simulink model "obs_servo_reduced"  (R2022a)
settings: Solver=VariableStepAuto  StartTime=0.0  StopTime=20  RelTol=1e-3
values from neighbouring files (symbols this model uses):
  A = [0 0 0 1 0 0 ... (first row only)    [main.m]
  Aroi = inv(Aro)    [main.m]
  B = [0 0 ... (first row only)    [main.m]
  C = [1 0 0 0 0 0 ... (first row only)    [main.m]
  D1 = [-3.6,0,0 ... (first row only)    [main.m]
  Eo = Tr*B    [main.m]
  Go = eye(3)    [main.m]
  ka5 = real(inv(R)*Ba5'*P2)    [main.m]
  ysp = -0.1*C*inv(A)*B*[-0.5+(a-b)/20;0.1+(b-c/(a+d+10))]    [main.m]
settings Model: Creator=wyton  LastModifiedBy=dzsgy
settings SolverCC: AlgebraicLoopSolver=TrustRegion
settings DebuggingCC: UnconnectedInputMsg=warning  UnconnectedOutputMsg=warning  UnconnectedLineMsg=warning  SFMachineParentedDataDiag=warning

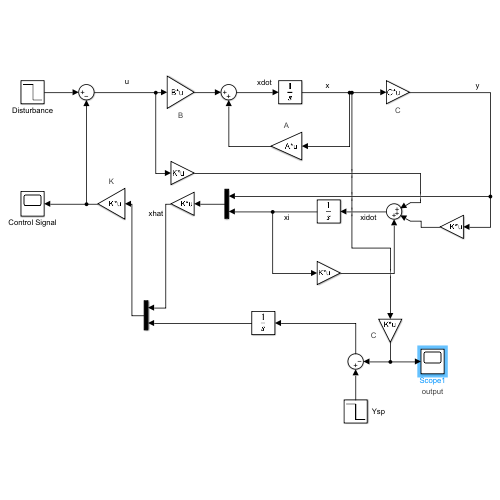
[thumbnail: Simulink's stored preview of the top-level diagram]
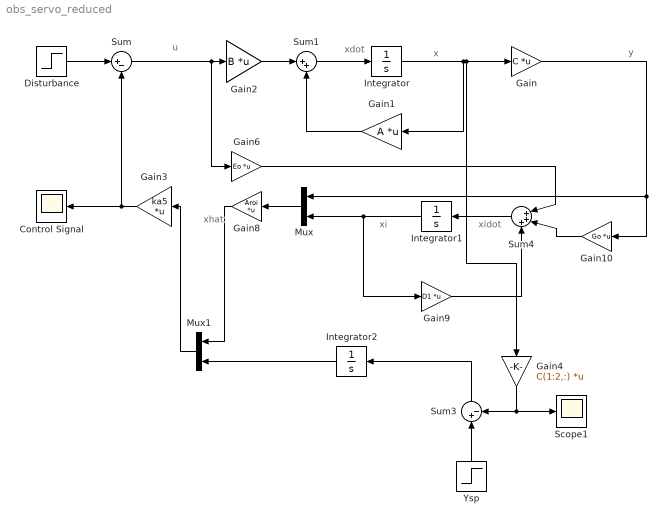
== system obs_servo_reduced ==
  note: xi
  note: xidot
  note: y
  note: xhat
  note: u
  note: xdot
  note: x
  Control Signal : Scope
  Disturbance : Step  Time=10  After=[-1,1]  SampleTime=0
  Gain : Gain  Gain=C  Multiplication=Matrix(K*u)
      settings: AttributesFormatString=C
  Gain1 : Gain  Gain=A  Multiplication=Matrix(K*u)
      settings: AttributesFormatString=A
  Gain10 : Gain  Gain=Go  Multiplication=Matrix(K*u)
  Gain2 : Gain  Tag=B  Gain=B  Multiplication=Matrix(K*u)
      settings: AttributesFormatString=B
  Gain3 : Gain  Gain=ka5  Multiplication=Matrix(K*u)
      settings: AttributesFormatString=K
  Gain4 : Gain  Gain=C(1:2,:)  Multiplication=Matrix(K*u)
      settings: AttributesFormatString=C
  Gain6 : Gain  Gain=Eo  Multiplication=Matrix(K*u)
  Gain8 : Gain  Gain=Aroi  Multiplication=Matrix(K*u)
  Gain9 : Gain  Gain=D1  Multiplication=Matrix(K*u)
  Integrator : Integrator
  Integrator1 : Integrator
  Integrator2 : Integrator
  Mux : Mux  Inputs=2
  Mux1 : Mux  Inputs=2
  Scope1 : Scope
      settings: AttributesFormatString=output
  Sum : Sum  Inputs=|+-
  Sum1 : Sum  Inputs=|++
  Sum3 : Sum  Inputs=|+-
  Sum4 : Sum  Inputs=|+++
  Ysp : Step  Time=0  After=[ysp(1),ysp(2)]  SampleTime=0
  wires:
  Sum/1 -> Gain6/1, Gain2/1
  Sum1/1 -> Integrator/1
  Gain2/1 -> Sum1/1
  Integrator/1 -> Gain4/1, Gain/1, Gain1/1
  Gain1/1 -> Sum1/2
  Gain3/1 -> Control Signal/1, Sum/2
  Mux/1 -> Gain8/1
  Integrator1/1 -> Gain9/1, Mux/2
  Sum4/1 -> Integrator1/1
  Gain9/1 -> Sum4/3
  Gain10/1 -> Sum4/2
  Gain6/1 -> Sum4/1
  Gain8/1 -> Mux1/1
  Ysp/1 -> Sum3/1
  Integrator2/1 -> Mux1/2
  Gain/1 -> Gain10/1, Mux/1
  Sum3/1 -> Integrator2/1
  Mux1/1 -> Gain3/1
  Disturbance/1 -> Sum/1
  Gain4/1 -> Scope1/1, Sum3/2
